simulink model "drone_model"  (R2025b)
settings: Solver=VariableStepAuto  StartTime=0.0  StopTime=12  RelTol=1e-3
values from neighbouring files (symbols this model uses):
  g = 9.81    [globals.m]
  Ixb = 0.0033    [globals.m]
  Iyb = 0.0033    [globals.m]
  Izb = 0.0058    [globals.m]
  m = 0.547    [globals.m]
  pitch_Kd = 1    [globals.m]
  pitch_Ki = 1    [globals.m]
  pitch_Kp = 1    [globals.m]
  roll_Kd = 1    [globals.m]
  roll_Ki = 1    [globals.m]
  roll_Kp = 1    [globals.m]
  yaw_Kd = 1    [globals.m]
  yaw_Ki = 1    [globals.m]
  yaw_Kp = 1    [globals.m]
  z_Kd = 1    [globals.m]
  z_Ki = 1    [globals.m]
  z_Kp = 1    [globals.m]
settings Model: Creator=JaiWillems  LastModifiedBy=JaiWillems

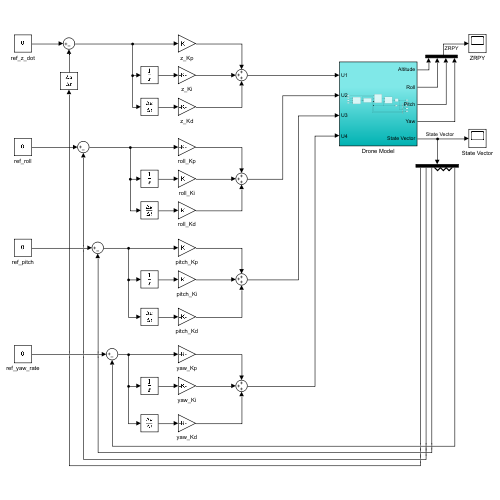
[thumbnail: Simulink's stored preview of the top-level diagram]
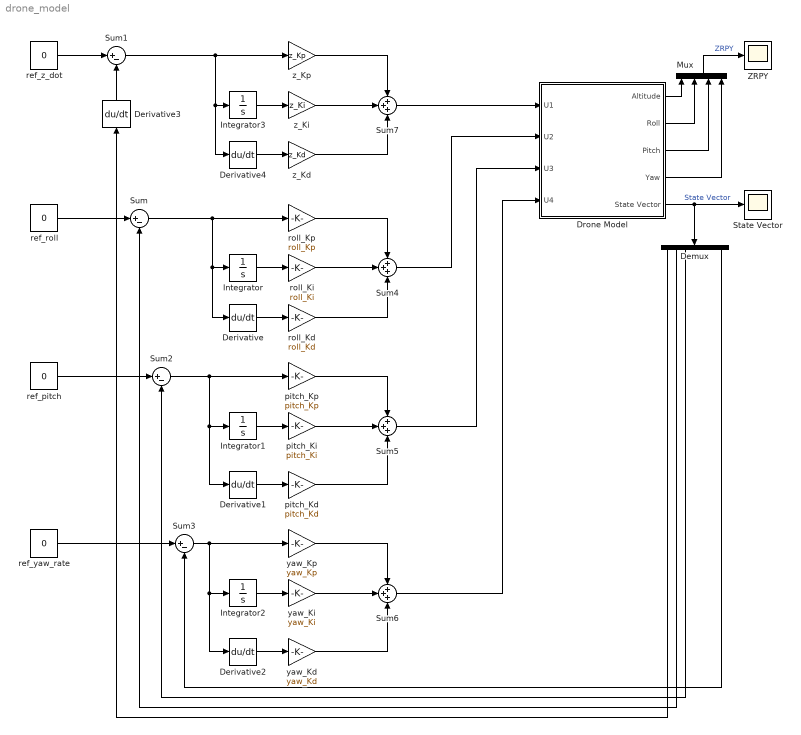
== system drone_model ==
  Demux : Demux  Outputs=7
  Derivative{,1..4} (5 alike) : Derivative
  Drone Model : Subsystem
  Integrator{,1..3} (4 alike) : Integrator
  Mux : Mux
  State Vector : Scope
      settings: ActiveDisplayYMinimum=-375.08949208928635  ActiveDisplayYMaximum=58.51162706715975
  Sum{,1..3} (4 alike) : Sum  Inputs=|+-
  Sum{4..7} (4 alike) : Sum  Inputs=+++
  ZRPY : Scope
      settings: ActiveDisplayYMinimum=-1.3379095016755045  ActiveDisplayYMaximum=3.2576673176429
  pitch_Kd : Gain  Gain=pitch_Kd
  pitch_Ki : Gain  Gain=pitch_Ki
  pitch_Kp : Gain  Gain=pitch_Kp
  ref_pitch : Constant  Value=0
  ref_roll : Constant  Value=0
  ref_yaw_rate : Constant  Value=0
  ref_z_dot : Constant  Value=0
  roll_Kd : Gain  Gain=roll_Kd
  roll_Ki : Gain  Gain=roll_Ki
  roll_Kp : Gain  Gain=roll_Kp
  yaw_Kd : Gain  Gain=yaw_Kd
  yaw_Ki : Gain  Gain=yaw_Ki
  yaw_Kp : Gain  Gain=yaw_Kp
  z_Kd : Gain  Gain=z_Kd
  z_Ki : Gain  Gain=z_Ki
  z_Kp : Gain  Gain=z_Kp
  wires:
  ref_z_dot/1 -> Sum1/1
  ref_roll/1 -> Sum/1
  ref_pitch/1 -> Sum2/1
  ref_yaw_rate/1 -> Sum3/1
  Drone Model/5(State Vector) -> Demux/1, State Vector/1  "State Vector"
  Drone Model/1(Altitude) -> Mux/1
  Drone Model/2(Roll) -> Mux/2
  Drone Model/3(Pitch) -> Mux/3
  Drone Model/4(Yaw) -> Mux/4
  Mux/1 -> ZRPY/1  "ZRPY"
  Demux/2 -> Sum/2
  Demux/3 -> Sum2/2
  Demux/7 -> Sum3/2
  Sum/1 -> Derivative/1, Integrator/1, roll_Kp/1
  Integrator/1 -> roll_Ki/1
  roll_Ki/1 -> Sum4/2
  roll_Kp/1 -> Sum4/1
  roll_Kd/1 -> Sum4/3
  Sum4/1 -> Drone Model/2(U2)
  pitch_Kp/1 -> Sum5/1
  pitch_Kd/1 -> Sum5/3
  Integrator1/1 -> pitch_Ki/1
  pitch_Ki/1 -> Sum5/2
  Sum2/1 -> Derivative1/1, Integrator1/1, pitch_Kp/1
  Sum5/1 -> Drone Model/3(U3)
  Derivative/1 -> roll_Kd/1
  Derivative1/1 -> pitch_Kd/1
  Sum6/1 -> Drone Model/4(U4)
  yaw_Kp/1 -> Sum6/1
  Derivative2/1 -> yaw_Kd/1
  Integrator2/1 -> yaw_Ki/1
  Sum3/1 -> Derivative2/1, Integrator2/1, yaw_Kp/1
  yaw_Ki/1 -> Sum6/2
  yaw_Kd/1 -> Sum6/3
  Demux/1 -> Derivative3/1
  Derivative3/1 -> Sum1/2
  Sum1/1 -> z_Kp/1, Derivative4/1, Integrator3/1
  z_Kp/1 -> Sum7/1
  Sum7/1 -> Drone Model/1(U1)
  z_Kd/1 -> Sum7/3
  Integrator3/1 -> z_Ki/1
  Derivative4/1 -> z_Kd/1
  z_Ki/1 -> Sum7/2

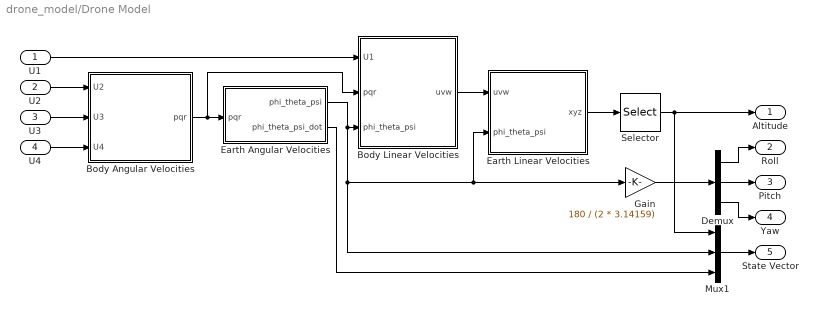
== system drone_model/Drone Model ==
  U1 : Inport
  U2 : Inport  Port=2
  U3 : Inport  Port=3
  U4 : Inport  Port=4
  Body Angular Velocities : Subsystem
  Body Linear Velocities : Subsystem
  Demux : Demux  Outputs=3
  Earth Angular Velocities : Subsystem
  Earth Linear Velocities : Subsystem
  Gain : Gain  Gain=180 / (2 * 3.14159)
  Mux1 : Mux  Inputs=3
  Selector : Selector  InputPortWidth=3  IndexOptions=Index vector (dialog)  Indices=3  OutputSizes=1
  Altitude : Outport
  Roll : Outport  Port=2
  Pitch : Outport  Port=3
  Yaw : Outport  Port=4
  State Vector : Outport  Port=5
  wires:
  Selector/1 -> Altitude/1, Mux1/1
  Body Linear Velocities/1(uvw) -> Earth Linear Velocities/1(uvw)
  Gain/1 -> Demux/1
  Body Angular Velocities/1(pqr) -> Body Linear Velocities/2(pqr), Earth Angular Velocities/1(pqr)
  Earth Angular Velocities/1(phi_theta_psi) -> Mux1/2, Earth Linear Velocities/2(phi_theta_psi), Gain/1, Body Linear Velocities/3(phi_theta_psi)
  Earth Linear Velocities/1(xyz) -> Selector/1
  Earth Angular Velocities/2(phi_theta_psi_dot) -> Mux1/3
  U4/1 -> Body Angular Velocities/3(U4)
  U2/1 -> Body Angular Velocities/1(U2)
  U3/1 -> Body Angular Velocities/2(U3)
  U1/1 -> Body Linear Velocities/1(U1)
  Mux1/1 -> State Vector/1
  Demux/2 -> Pitch/1
  Demux/1 -> Roll/1
  Demux/3 -> Yaw/1

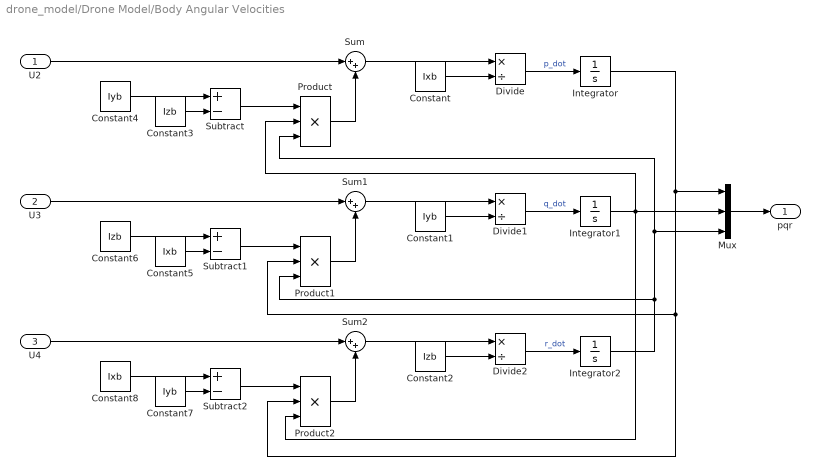
== system drone_model/Drone Model/Body Angular Velocities ==
  U2 : Inport
  U3 : Inport  Port=2
  U4 : Inport  Port=3
  Constant : Constant  Value=Ixb
  Constant1 : Constant  Value=Iyb
  Constant2 : Constant  Value=Izb
  Constant3 : Constant  Value=Izb
  Constant4 : Constant  Value=Iyb
  Constant5 : Constant  Value=Ixb
  Constant6 : Constant  Value=Izb
  Constant7 : Constant  Value=Iyb
  Constant8 : Constant  Value=Ixb
  Divide : Product  Inputs=*/
  Divide1 : Product  Inputs=*/
  Divide2 : Product  Inputs=*/
  Integrator : Integrator
  Integrator1 : Integrator
  Integrator2 : Integrator
  Mux : Mux  Inputs=3
  Product : Product  Inputs=3
  Product1 : Product  Inputs=3
  Product2 : Product  Inputs=3
  Subtract : Sum  Inputs=+-
  Subtract1 : Sum  Inputs=+-
  Subtract2 : Sum  Inputs=+-
  Sum : Sum  Inputs=|++
  Sum1 : Sum  Inputs=|++
  Sum2 : Sum  Inputs=|++
  pqr : Outport
  wires:
  Integrator/1 -> Mux/1, Product1/2, Product2/2
  Product/1 -> Sum/2
  U2/1 -> Sum/1
  Divide/1 -> Integrator/1  "p_dot"
  Sum/1 -> Divide/1
  Constant/1 -> Divide/2
  Integrator1/1 -> Product/2, Mux/2, Product2/3
  Integrator2/1 -> Product1/3, Product/3, Mux/3
  Divide1/1 -> Integrator1/1  "q_dot"
  Divide2/1 -> Integrator2/1  "r_dot"
  Constant1/1 -> Divide1/2
  Constant2/1 -> Divide2/2
  Sum1/1 -> Divide1/1
  U3/1 -> Sum1/1
  Sum2/1 -> Divide2/1
  U4/1 -> Sum2/1
  Product1/1 -> Sum1/2
  Product2/1 -> Sum2/2
  Subtract1/1 -> Product1/1
  Subtract2/1 -> Product2/1
  Constant3/1 -> Subtract/2
  Constant4/1 -> Subtract/1
  Constant5/1 -> Subtract1/2
  Constant6/1 -> Subtract1/1
  Constant7/1 -> Subtract2/2
  Constant8/1 -> Subtract2/1
  Subtract/1 -> Product/1
  Mux/1 -> pqr/1

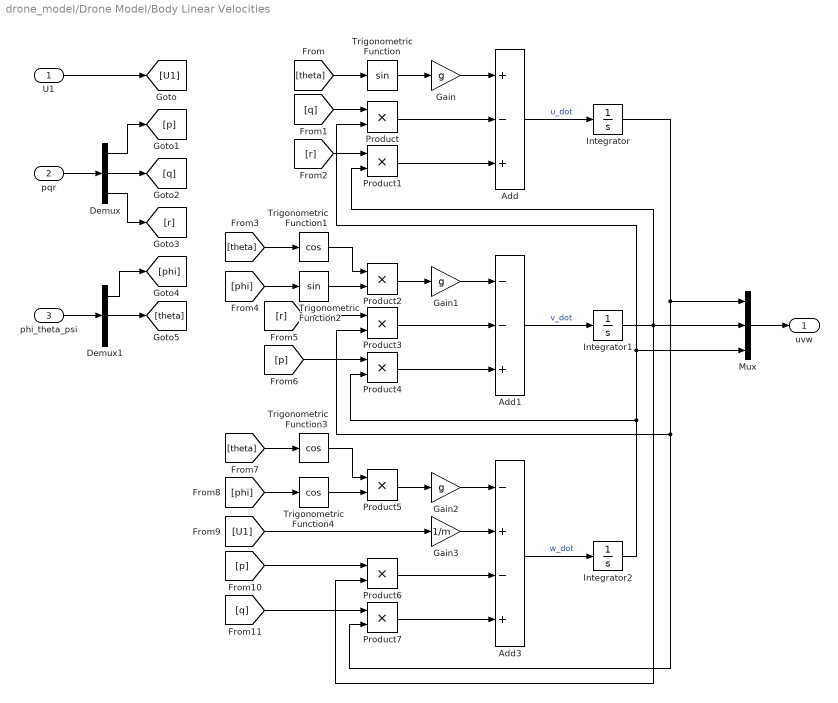
== system drone_model/Drone Model/Body Linear Velocities ==
  U1 : Inport
  pqr : Inport  Port=2
  phi_theta_psi : Inport  Port=3
  Add : Sum  Inputs=+-+
  Add1 : Sum  Inputs=--+
  Add3 : Sum  Inputs=-+-+
  Demux : Demux  Outputs=3
  Demux1 : Demux  Outputs=3
  Gain : Gain  Gain=g
  Gain1 : Gain  Gain=g
  Gain2 : Gain  Gain=g
  Gain3 : Gain  Gain=1/m
  Integrator : Integrator
  Integrator1 : Integrator
  Integrator2 : Integrator
  Mux : Mux  Inputs=3
  Product{,1..7} (8 alike) : Product
  Trigonometric Function : Trigonometry
  Trigonometric Function1 : Trigonometry  Operator=cos
  Trigonometric Function2 : Trigonometry
  Trigonometric Function3 : Trigonometry  Operator=cos
  Trigonometric Function4 : Trigonometry  Operator=cos
  uvw : Outport
  wires:
  Trigonometric Function2/1 -> Product2/2
  Add1/1 -> Integrator1/1  "v_dot"
  Product1/1 -> Add/3
  Trigonometric Function4/1 -> Product5/2
  Trigonometric Function3/1 -> Product5/1
  Integrator1/1 -> Product1/2, Mux/2, Product6/2
  Integrator2/1 -> Product/2, Mux/3, Product4/2
  Trigonometric Function1/1 -> Product2/1
  Product2/1 -> Gain1/1
  Product5/1 -> Gain2/1
  Product/1 -> Add/2
  Integrator/1 -> Mux/1, Product3/2, Product7/2
  Trigonometric Function/1 -> Gain/1
  Add/1 -> Integrator/1  "u_dot"
  Gain/1 -> Add/1
  Add3/1 -> Integrator2/1  "w_dot"
  Gain1/1 -> Add1/1
  Product4/1 -> Add1/3
  Product3/1 -> Add1/2
  U1/1 -> [U1]
  [theta] -> Trigonometric Function/1
  [q] -> Product/1
  [r] -> Product1/1
  [theta] -> Trigonometric Function1/1
  [phi] -> Trigonometric Function2/1
  [r] -> Product3/1
  [p] -> Product4/1
  Gain2/1 -> Add3/1
  [theta] -> Trigonometric Function3/1
  [phi] -> Trigonometric Function4/1
  Gain3/1 -> Add3/2
  [U1] -> Gain3/1
  Product6/1 -> Add3/3
  Product7/1 -> Add3/4
  [p] -> Product6/1
  [q] -> Product7/1
  Demux/2 -> [q]
  Demux/1 -> [p]
  Demux/3 -> [r]
  pqr/1 -> Demux/1
  Mux/1 -> uvw/1
  Demux1/1 -> [phi]
  Demux1/2 -> [theta]
  phi_theta_psi/1 -> Demux1/1

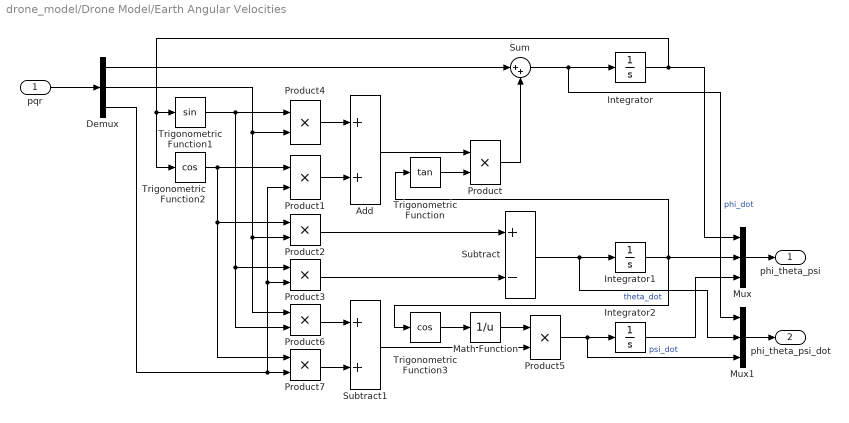
== system drone_model/Drone Model/Earth Angular Velocities ==
  pqr : Inport
  Add : Sum
  Demux : Demux  Outputs=3
  Integrator : Integrator
  Integrator1 : Integrator
  Integrator2 : Integrator
  Math Function : Math  Operator=reciprocal
  Mux : Mux  Inputs=3
  Mux1 : Mux  Inputs=3
  Product{,1..7} (8 alike) : Product
  Subtract : Sum  Inputs=+-
  Subtract1 : Sum
  Sum : Sum  Inputs=|++
  Trigonometric Function : Trigonometry  Operator=tan
  Trigonometric Function1 : Trigonometry
  Trigonometric Function2 : Trigonometry  Operator=cos
  Trigonometric Function3 : Trigonometry  Operator=cos
  phi_theta_psi : Outport
  phi_theta_psi_dot : Outport  Port=2
  wires:
  Integrator/1 -> Mux/1, Trigonometric Function2/1, Trigonometric Function1/1
  Integrator1/1 -> Trigonometric Function/1, Mux/2, Trigonometric Function3/1
  Sum/1 -> Integrator/1, Mux1/1  "phi_dot"
  Demux/2 -> Product6/1, Product2/2, Product4/2
  Demux/3 -> Product7/2, Product1/2, Product3/2
  Subtract/1 -> Integrator1/1, Mux1/2  "theta_dot"
  Product2/1 -> Subtract/1
  Product3/1 -> Subtract/2
  Demux/1 -> Sum/1
  Add/1 -> Product/1
  Trigonometric Function/1 -> Product/2
  Product/1 -> Sum/2
  Product1/1 -> Add/2
  Product4/1 -> Add/1
  Trigonometric Function1/1 -> Product6/2, Product3/1, Product4/1
  Trigonometric Function2/1 -> Product2/1, Product7/1, Product1/1
  Math Function/1 -> Product5/1
  Product5/1 -> Integrator2/1, Mux1/3  "psi_dot"
  Product7/1 -> Subtract1/2
  Product6/1 -> Subtract1/1
  Trigonometric Function3/1 -> Math Function/1
  Subtract1/1 -> Product5/2
  pqr/1 -> Demux/1
  Mux/1 -> phi_theta_psi/1
  Integrator2/1 -> Mux/3
  Mux1/1 -> phi_theta_psi_dot/1

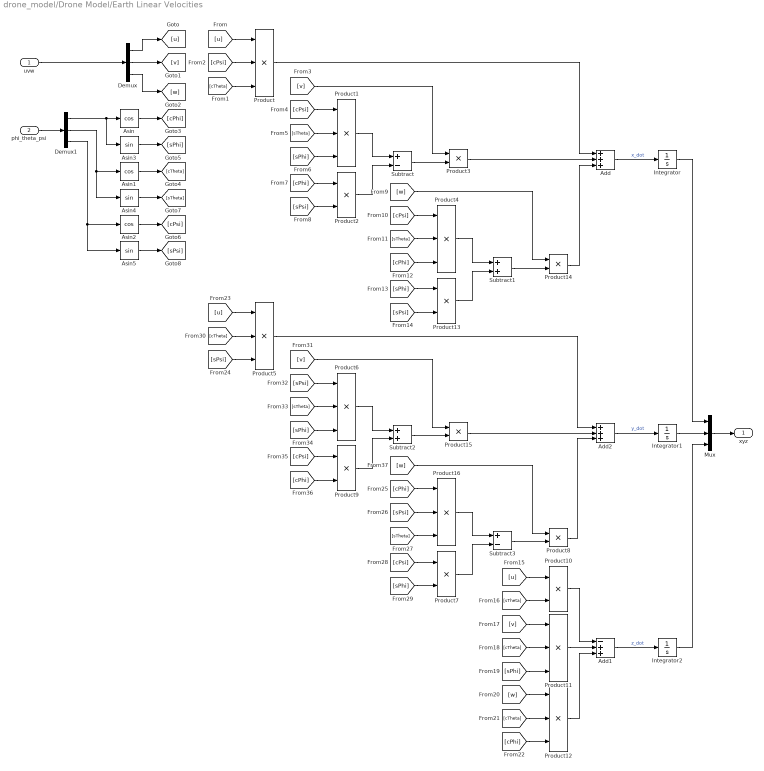
== system drone_model/Drone Model/Earth Linear Velocities ==
  uvw : Inport
  phi_theta_psi : Inport  Port=2
  Add : Sum  Inputs=+++
  Add1 : Sum  Inputs=-++
  Add2 : Sum  Inputs=+++
  Asin : Trigonometry  Operator=cos
  Asin1 : Trigonometry  Operator=cos
  Asin2 : Trigonometry  Operator=cos
  Asin3 : Trigonometry
  Asin4 : Trigonometry
  Asin5 : Trigonometry
  Demux : Demux  Outputs=3
  Demux1 : Demux  Outputs=3
  Integrator : Integrator
  Integrator1 : Integrator
  Integrator2 : Integrator
  Mux : Mux  Inputs=3
  Product{,1,4..6,11..12,16} (8 alike) : Product  Inputs=3
  Product{2..3,7..10,13..15} (9 alike) : Product
  Subtract : Sum  Inputs=+-
  Subtract1 : Sum
  Subtract2 : Sum
  Subtract3 : Sum  Inputs=+-
  xyz : Outport
  wires:
  Add/1 -> Integrator/1  "x_dot"
  Add2/1 -> Integrator1/1  "y_dot"
  Add1/1 -> Integrator2/1  "z_dot"
  Asin/1 -> [cPhi]
  Asin3/1 -> [sPhi]
  Asin1/1 -> [cTheta]
  Asin4/1 -> [sTheta]
  Asin2/1 -> [cPsi]
  Asin5/1 -> [sPsi]
  Demux1/2 -> Asin1/1, Asin4/1
  Demux1/3 -> Asin2/1, Asin5/1
  [cPsi] -> Product/2
  [u] -> Product/1
  [cTheta] -> Product/3
  [cPsi] -> Product1/1
  [sTheta] -> Product1/2
  [sPhi] -> Product1/3
  [cPhi] -> Product2/1
  [sPsi] -> Product2/2
  Product1/1 -> Subtract/1
  Product2/1 -> Subtract/2
  Subtract/1 -> Product3/2
  [v] -> Product3/1
  Product/1 -> Add/1
  Product3/1 -> Add/2
  Product14/1 -> Add/3
  Product4/1 -> Subtract1/1
  Product13/1 -> Subtract1/2
  [sPsi] -> Product13/2
  [w] -> Product14/1
  Subtract1/1 -> Product14/2
  [sTheta] -> Product4/2
  [sPhi] -> Product13/1
  [cPsi] -> Product4/1
  [cPhi] -> Product4/3
  [u] -> Product10/1
  [sTheta] -> Product10/2
  [v] -> Product11/1
  [cTheta] -> Product11/2
  [sPhi] -> Product11/3
  [w] -> Product12/1
  [cTheta] -> Product12/2
  [cPhi] -> Product12/3
  Product10/1 -> Add1/1
  Product11/1 -> Add1/2
  Product12/1 -> Add1/3
  [cTheta] -> Product5/2
  Product6/1 -> Subtract2/1
  [cPhi] -> Product9/2
  [v] -> Product15/1
  Product15/1 -> Add2/2
  Product8/1 -> Add2/3
  Product5/1 -> Add2/1
  Subtract2/1 -> Product15/2
  [sPsi] -> Product5/3
  [u] -> Product5/1
  [sTheta] -> Product16/3
  Product7/1 -> Subtract3/2
  Product16/1 -> Subtract3/1
  [cPhi] -> Product16/1
  Product9/1 -> Subtract2/2
  Subtract3/1 -> Product8/2
  [sPsi] -> Product16/2
  [cPsi] -> Product7/1
  [sPsi] -> Product6/1
  [cPsi] -> Product9/1
  [sTheta] -> Product6/2
  [w] -> Product8/1
  [sPhi] -> Product6/3
  [sPhi] -> Product7/2
  uvw/1 -> Demux/1
  Demux/1 -> [u]
  Demux/2 -> [v]
  Demux/3 -> [w]
  Integrator1/1 -> Mux/2
  Mux/1 -> xyz/1
  Integrator/1 -> Mux/1
  Integrator2/1 -> Mux/3
  phi_theta_psi/1 -> Demux1/1
  Demux1/1 -> Asin3/1, Asin/1
